simulink model "CartPendReal"  (R2015a)
settings: Solver=ode5  SolverMode=SingleTasking  StartTime=0.0  StopTime=inf  FixedStep=Ts  RelTol=1e-3  AbsTol=1e-6
values from neighbouring files (symbols this model uses):
  g = 9.81    [CartPendParams.mat]
  Jp = 0.00800173441225    [CartPendParams.mat]
  lpo = 0.20854    [CartPendParams.mat]
  lpwo = 0.455840449763    [CartPendParams.mat]
  mps = 0.0417185657763    [CartPendParams.mat]
  mpw = 0.0272036144897    [CartPendParams.mat]
  Ts = 0.01    [CartPendParams.mat]
  x0 = [0 3.14159265359 0 0]    [CartPendParams.mat]
undefined symbols (not defined in the file or in its folder): B1, B2, K, W1, W2
undefined symbols (not defined in the file): RTDAC4PCIBaseAddress
libraries: simulink x1
settings Model: SimulationMode=external  CovHtmlReporting=off  ExtModeTrigDuration=12000  ExtModeTrigLevel=0.400000  Creator=jims  LastModifiedBy=Student
settings DataIOCC: ExternalInput=[]  InitialState=[]  LimitDataPoints=off  MaxDataPoints=5000  SignalLoggingSaveFormat=ModelDataLogs  SaveOutput=off  SaveTime=off  SignalLoggingName=sigsOut
settings OptimizationCC: BooleanDataType=off  ExpressionDepthLimit=2147483647  InitFltsAndDblsToZero=on
settings DebuggingCC: SaveWithParameterizedLinksMsg=none  UnderspecifiedInitializationDetection=Classic  MergeDetectMultiDrivingBlocksExec=none  SignalResolutionControl=TryResolveAllWithWarning  MultiTaskDSMMsg=warning  MultiTaskCondExecSysMsg=none  IntegerOverflowMsg=none  FcnCallInpInsideContextMsg=EnableAllAsWarning  StateNameClashWarn=warning  IntegerSaturationMsg=none
settings HardwareCC: ProdBitPerLong=64  ProdBitPerPointer=64  ProdIntDivRoundTo=Zero  ProdEndianess=LittleEndian  ProdWordSize=64  ProdHWDeviceType=Intel->x86-64  TargetBitPerLong=64  TargetBitPerPointer=64  TargetIntDivRoundTo=Zero  TargetEndianess=LittleEndian  TargetWordSize=64  TargetHWDeviceType=Intel->x86-64
settings RTWCC: SystemTargetFile=rtwin.tlc  TemplateMakefile=RTDAC_win.tmf  Description=Real-Time Windows Target
settings RTWinTargetCC: TargetFcnLib=ansi_tfl_tmw.mat  TargetPreCompLibLocation=C:\Program Files\MATLAB\R2015aSP1\toolbox\sldrt\lib\win64  ModelReferenceCompliant=off  CompOptLevelCompliant=off

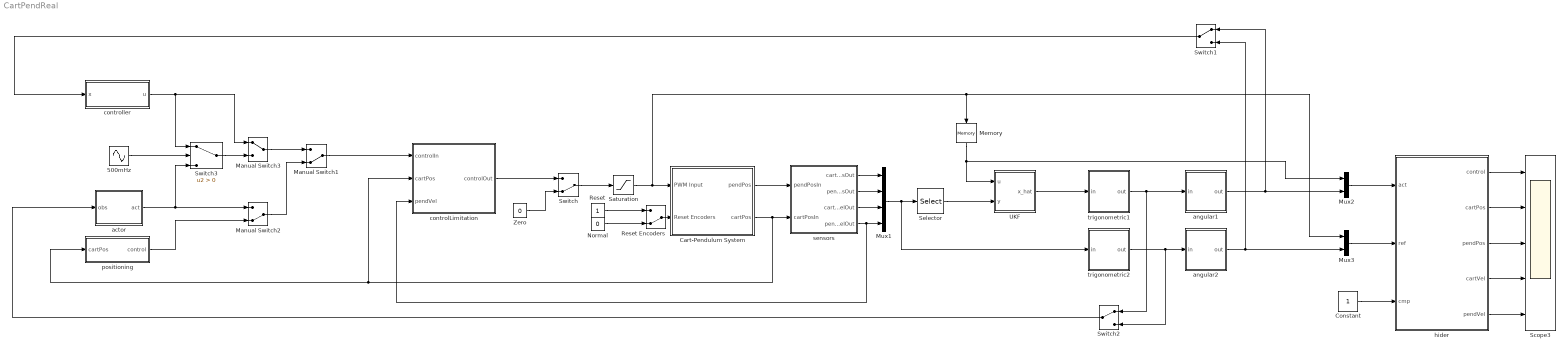
== system CartPendReal ==
  500mHz : Sin  Frequency=pi  SampleTime=Ts
  Cart-Pendulum System : Subsystem  mask{BaseAddress=RTDAC4PCIBaseAddress(-1,-1), T0=Ts}
      mask prompts: BaseAddress "Base Address:"; T0 "Sampling Period:"
      mask Display: plot( [0.725 0.725], [1.05 0.375], 0.725+0.05*sin([0:0.5:7]), 0.325+0.05*cos([0:0.5:7]), [-0.3 -0.3], [-0.3 -0.3], [1.8 1.8], [1.8 1.8], [0.1 1.4], [0.95 0.95], [0.1 1.4], [0.92 0.92], [0.65 0.8], [1 1], [0.65 0.8], [1.1 1.1], [0.65 0.65], [1.1 1], [0.8 0.8], [1 1.1] )
  Constant : Constant
  Manual Switch1 : ManualSwitch  CurrentSetting=0
  Manual Switch2 : ManualSwitch  CurrentSetting=0
  Manual Switch3 : ManualSwitch
  Memory : Memory
  Mux1 : Mux
  Mux2 : Mux  Inputs=2
  Mux3 : Mux  Inputs=2
  Normal : Constant  Value=0
  Reset : Constant
  Reset Encoders : ManualSwitch  CurrentSetting=0
  Saturation : Saturate
  Scope3 : Scope  NumInputPorts=5
      settings: TimeRange=15  YMin=-0.6~-1~-3.141592653589793~-5~-12  YMax=0.6~1~3.141592653589793~5~12  SampleInput=on  SampleTime=Ts  ScrollMode=on
  Selector : Selector  InputPortWidth=4  Indices=[1 2]
  Switch : ManualSwitch  CurrentSetting=0
  Switch1 : ManualSwitch
  Switch2 : ManualSwitch
  Switch3 : Switch  Criteria=u2 > Threshold
  UKF : Subsystem
  Zero : Constant  Value=0
  actor : MATLAB Function  TreatAsAtomicUnit=on  SystemSampleTime=Ts
  angular1 : Subsystem
  angular2 : Subsystem
  controlLimitation : Subsystem
  controller : Subsystem
  hider : Subsystem
  positioning : Subsystem
  sensors : Subsystem  mask(PENDULUM Output){T0=Ts}
      mask prompts: T0 "Sample Time"
      mask help: PCL-812 PG Device Driver
  trigonometric1 : Subsystem
  trigonometric2 : Subsystem
  wires:
  actor/1(act) -> Manual Switch2/1, Switch3/3
  Switch/1 -> Saturation/1
  Reset Encoders/1 -> Cart-Pendulum System/2(Reset Encoders)
  Reset/1 -> Reset Encoders/1
  Normal/1 -> Reset Encoders/2
  sensors/4(pendVelOut) -> Mux1/4, controlLimitation/3(pendVel)
  sensors/1(cartPosOut) -> Mux1/1
  sensors/2(pendPosOut) -> Mux1/2
  sensors/3(cartVelOut) -> Mux1/3
  Constant/1 -> hider/3(cmp)
  Zero/1 -> Switch/2
  Saturation/1 -> Memory/1, Mux3/1, Cart-Pendulum System/1(PWM Input)
  Mux1/1 -> Selector/1, trigonometric2/1(in)
  hider/5(pendVel) -> Scope3/5
  Selector/1 -> UKF/2(y)
  Mux3/1 -> hider/2(ref)
  Mux2/1 -> hider/1(act)
  UKF/1(x_hat) -> trigonometric1/1(in)
  Cart-Pendulum System/1(pendPos) -> sensors/1(pendPosIn)
  trigonometric1/1(out) -> angular1/1(in), Switch2/1
  trigonometric2/1(out) -> Switch2/2, angular2/1(in)
  positioning/1(control) -> Manual Switch2/2
  Manual Switch2/1 -> Manual Switch1/2
  controller/1(u) -> Manual Switch3/1, Switch3/1
  angular1/1(out) -> Mux2/2, Switch1/1
  angular2/1(out) -> Switch1/2, Mux3/2
  hider/1(control) -> Scope3/1
  hider/2(cartPos) -> Scope3/2
  hider/3(pendPos) -> Scope3/3
  hider/4(cartVel) -> Scope3/4
  500mHz/1 -> Switch3/2
  Switch3/1 -> Manual Switch3/2
  Switch2/1 -> actor/1(obs)
  Manual Switch3/1 -> Manual Switch1/1
  Memory/1 -> UKF/1(u), Mux2/1
  controlLimitation/1(controlOut) -> Switch/1
  Cart-Pendulum System/2(cartPos) -> controlLimitation/2(cartPos), positioning/1(cartPos), sensors/2(cartPosIn)
  Switch1/1 -> controller/1(x)
  Manual Switch1/1 -> controlLimitation/1(controlIn)

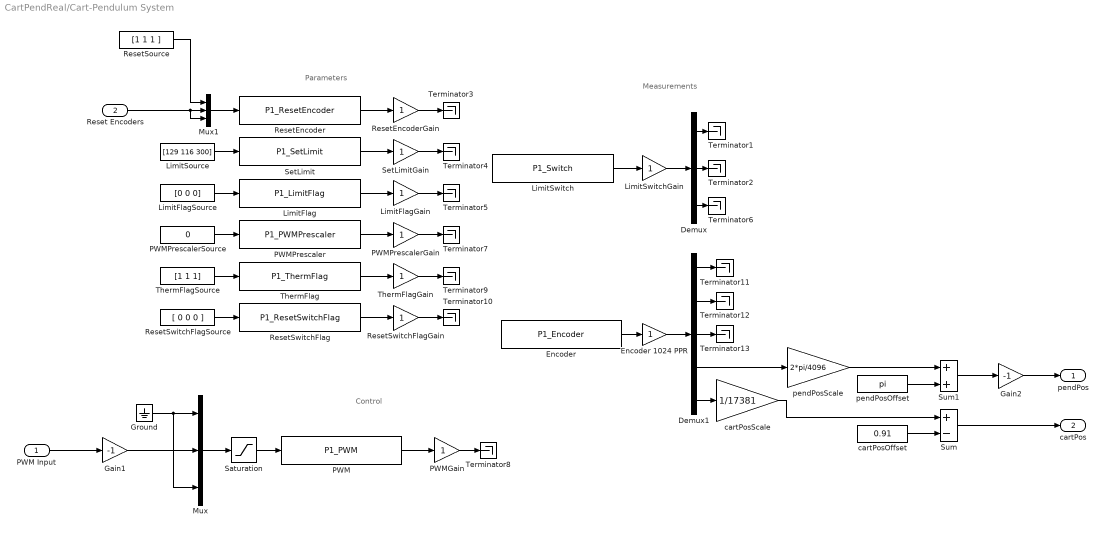
== system CartPendReal/Cart-Pendulum System ==
  note: Measurements
  note: Control
  note: Parameters
  PWM Input : Inport
  Reset Encoders : Inport  Port=2
  Demux : Demux  Outputs=3
  Demux1 : Demux  Outputs=5
  Encoder : S-Function  FunctionName=P1_Encoder  Parameters=BaseAddress, T0
  Encoder 1024 PPR : Gain  SaturateOnIntegerOverflow=on  OutDataTypeStr=Inherit: Same as input  ParamDataTypeStr=Inherit: Same as input
  Gain1 : Gain  Gain=-1
  Gain2 : Gain  Gain=-1
  Ground : Ground
  LimitFlag : S-Function  FunctionName=P1_LimitFlag  Parameters=BaseAddress, T0
  LimitFlagGain : Gain  SaturateOnIntegerOverflow=on  OutDataTypeStr=Inherit: Same as input  ParamDataTypeStr=Inherit: Same as input
  LimitFlagSource : Constant  Value=[0 0 0]
  LimitSource : Constant  Value=[129 116 300]
  LimitSwitch : S-Function  FunctionName=P1_Switch  Parameters=BaseAddress, T0
  LimitSwitchGain : Gain  SaturateOnIntegerOverflow=on  OutDataTypeStr=Inherit: Same as input  ParamDataTypeStr=Inherit: Same as input
  Mux : Mux  Inputs=3
  Mux1 : Mux  Inputs=[3 1 1]
  PWM : S-Function  FunctionName=P1_PWM  Parameters=BaseAddress, T0
  PWMGain : Gain  SaturateOnIntegerOverflow=on  OutDataTypeStr=Inherit: Same as input  ParamDataTypeStr=Inherit: Same as input
  PWMPrescaler : S-Function  FunctionName=P1_PWMPrescaler  Parameters=BaseAddress, T0
  PWMPrescalerGain : Gain  SaturateOnIntegerOverflow=on  OutDataTypeStr=Inherit: Same as input  ParamDataTypeStr=Inherit: Same as input
  PWMPrescalerSource : Constant  Value=0
  ResetEncoder : S-Function  FunctionName=P1_ResetEncoder  Parameters=BaseAddress, T0
  ResetEncoderGain : Gain  SaturateOnIntegerOverflow=on  OutDataTypeStr=Inherit: Same as input  ParamDataTypeStr=Inherit: Same as input
  ResetSource : Constant  Value=[1 1 1 ]
  "ResetSwitchFlag " : S-Function  FunctionName=P1_ResetSwitchFlag  Parameters=BaseAddress, T0
  ResetSwitchFlagGain : Gain  SaturateOnIntegerOverflow=on  OutDataTypeStr=Inherit: Same as input  ParamDataTypeStr=Inherit: Same as input
  ResetSwitchFlagSource : Constant  Value=[ 0 0 0 ]
  Saturation : Saturate
  SetLimit : S-Function  FunctionName=P1_SetLimit  Parameters=BaseAddress, T0
  SetLimitGain : Gain  SaturateOnIntegerOverflow=on  OutDataTypeStr=Inherit: Same as input  ParamDataTypeStr=Inherit: Same as input
  Sum : Sum  Inputs=+-  SaturateOnIntegerOverflow=on  InputSameDT=on  OutDataTypeStr=Inherit: Same as first input
  Sum1 : Sum  SaturateOnIntegerOverflow=on  InputSameDT=on  OutDataTypeStr=Inherit: Same as first input
  Terminator{1..13} (13 alike) : Terminator
  "ThermFlag " : S-Function  FunctionName=P1_ThermFlag  Parameters=BaseAddress, T0
  ThermFlagGain : Gain  SaturateOnIntegerOverflow=on  OutDataTypeStr=Inherit: Same as input  ParamDataTypeStr=Inherit: Same as input
  ThermFlagSource : Constant  Value=[1 1 1]
  cartPosOffset : Constant  Value=0.91
  cartPosScale : Gain  Gain=1/17381  OutDataTypeStr=Inherit: Same as input  ParamDataTypeStr=Inherit: Same as input
  pendPosOffset : Constant  Value=pi
  pendPosScale : Gain  Gain=2*pi/4096  OutDataTypeStr=Inherit: Same as input  ParamDataTypeStr=Inherit: Same as input
  pendPos : Outport
  cartPos : Outport  Port=2
  wires:
  Demux1/1 -> Terminator11/1
  Demux1/2 -> Terminator12/1
  Demux1/3 -> Terminator13/1
  Demux/3 -> Terminator6/1
  Demux/2 -> Terminator2/1
  Demux/1 -> Terminator1/1
  LimitSwitchGain/1 -> Demux/1
  LimitSwitch/1 -> LimitSwitchGain/1
  Ground/1 -> Mux/1, Mux/3
  PWM Input/1 -> Gain1/1
  ResetSwitchFlagGain/1 -> Terminator10/1
  ThermFlagGain/1 -> Terminator9/1
  PWMPrescalerGain/1 -> Terminator7/1
  LimitFlagGain/1 -> Terminator5/1
  SetLimitGain/1 -> Terminator4/1
  ResetEncoderGain/1 -> Terminator3/1
  ResetSwitchFlagSource/1 -> "ResetSwitchFlag "/1
  ThermFlagSource/1 -> "ThermFlag "/1
  PWMPrescalerSource/1 -> PWMPrescaler/1
  LimitFlagSource/1 -> LimitFlag/1
  LimitSource/1 -> SetLimit/1
  "ResetSwitchFlag "/1 -> ResetSwitchFlagGain/1
  "ThermFlag "/1 -> ThermFlagGain/1
  PWMPrescaler/1 -> PWMPrescalerGain/1
  LimitFlag/1 -> LimitFlagGain/1
  SetLimit/1 -> SetLimitGain/1
  ResetEncoder/1 -> ResetEncoderGain/1
  PWMGain/1 -> Terminator8/1
  PWM/1 -> PWMGain/1
  Mux/1 -> Saturation/1
  Saturation/1 -> PWM/1
  Encoder/1 -> Encoder 1024 PPR/1
  Encoder 1024 PPR/1 -> Demux1/1
  Mux1/1 -> ResetEncoder/1
  ResetSource/1 -> Mux1/1
  Reset Encoders/1 -> Mux1/2, Mux1/3
  pendPosScale/1 -> Sum1/1
  pendPosOffset/1 -> Sum1/2
  Gain1/1 -> Mux/2
  Sum1/1 -> Gain2/1
  Sum/1 -> cartPos/1
  Demux1/4 -> pendPosScale/1
  Gain2/1 -> pendPos/1
  Demux1/5 -> cartPosScale/1
  cartPosOffset/1 -> Sum/2
  cartPosScale/1 -> Sum/1

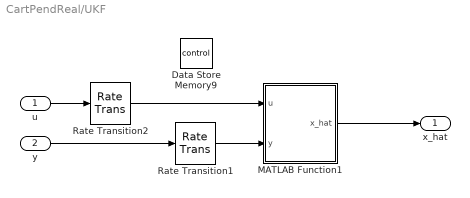
== system CartPendReal/UKF ==
  u : Inport
  y : Inport  Port=2
  Data Store Memory9 : DataStoreMemory  DataStoreName=control  ReadBeforeWriteMsg=warning  WriteAfterWriteMsg=warning  WriteAfterReadMsg=warning  OutDataTypeStr=double
  MATLAB Function1 : MATLAB Function  TreatAsAtomicUnit=on
  Rate Transition1 : RateTransition  X0=x0(1:2)  OutPortSampleTime=Ts
  Rate Transition2 : RateTransition  OutPortSampleTime=Ts
  x_hat : Outport
  wires:
  Rate Transition2/1 -> MATLAB Function1/1(u)
  Rate Transition1/1 -> MATLAB Function1/2(y)
  y/1 -> Rate Transition1/1
  MATLAB Function1/1(x_hat) -> x_hat/1
  u/1 -> Rate Transition2/1

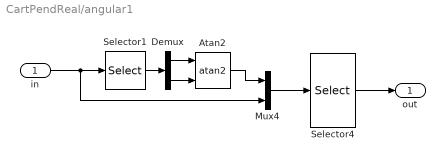
== system CartPendReal/angular1 ==
  in : Inport
  Atan2 : Trigonometry  Operator=atan2
  Demux : Demux  Outputs=2
  Mux4 : Mux  Inputs=2
  Selector1 : Selector  InputPortWidth=5  Indices=[2 3]
  Selector4 : Selector  InputPortWidth=6  Indices=[2 1 5 6]
  out : Outport
  wires:
  Demux/2 -> Atan2/2
  in/1 -> Mux4/2, Selector1/1
  Atan2/1 -> Mux4/1
  Demux/1 -> Atan2/1
  Mux4/1 -> Selector4/1
  Selector4/1 -> out/1
  Selector1/1 -> Demux/1

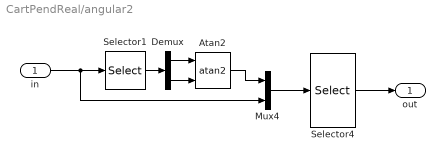
== system CartPendReal/angular2 ==
  in : Inport
  Atan2 : Trigonometry  Operator=atan2
  Demux : Demux  Outputs=2
  Mux4 : Mux  Inputs=2
  Selector1 : Selector  InputPortWidth=5  Indices=[2 3]
  Selector4 : Selector  InputPortWidth=6  Indices=[2 1 5 6]
  out : Outport
  wires:
  Demux/2 -> Atan2/2
  in/1 -> Mux4/2, Selector1/1
  Atan2/1 -> Mux4/1
  Demux/1 -> Atan2/1
  Mux4/1 -> Selector4/1
  Selector4/1 -> out/1
  Selector1/1 -> Demux/1

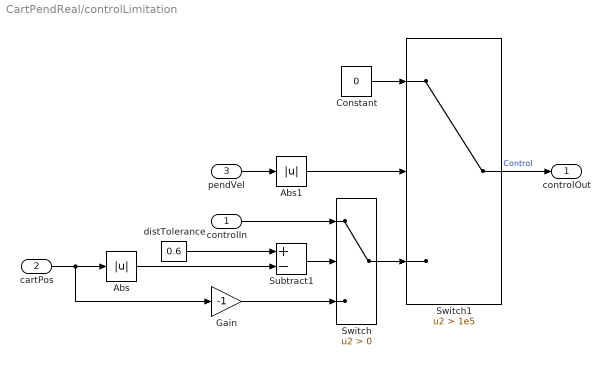
== system CartPendReal/controlLimitation ==
  controlIn : Inport
  cartPos : Inport  Port=2
  pendVel : Inport  Port=3
  Abs : Abs
  Abs1 : Abs
  Constant : Constant  Value=0
  Gain : Gain  Gain=-1
  Subtract1 : Sum  Inputs=+-
  Switch : Switch  Criteria=u2 > Threshold
  Switch1 : Switch  Criteria=u2 > Threshold  Threshold=1e5
  distTolerance : Constant  Value=0.6
  controlOut : Outport
  wires:
  controlIn/1 -> Switch/1
  distTolerance/1 -> Subtract1/1
  Switch1/1 -> controlOut/1  "Control"
  Subtract1/1 -> Switch/2
  Abs/1 -> Subtract1/2
  cartPos/1 -> Abs/1, Gain/1
  Gain/1 -> Switch/3
  pendVel/1 -> Abs1/1
  Abs1/1 -> Switch1/2
  Constant/1 -> Switch1/1
  Switch/1 -> Switch1/3

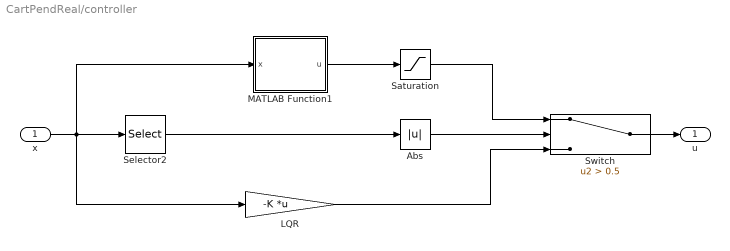
== system CartPendReal/controller ==
  x : Inport
  Abs : Abs
  LQR : Gain  Gain=-K  Multiplication=Matrix(K*u) (u vector)
  MATLAB Function1 : MATLAB Function  TreatAsAtomicUnit=on  SystemSampleTime=Ts
  Saturation : Saturate  UpperLimit=0.4  LowerLimit=-0.4
  Selector2 : Selector  InputPortWidth=4  Indices=[2]
  Switch : Switch  Criteria=u2 > Threshold  Threshold=0.5
  u : Outport
  wires:
  MATLAB Function1/1(u) -> Saturation/1
  Selector2/1 -> Abs/1
  Abs/1 -> Switch/2
  Switch/1 -> u/1
  x/1 -> LQR/1, Selector2/1, MATLAB Function1/1(x)
  LQR/1 -> Switch/3
  Saturation/1 -> Switch/1

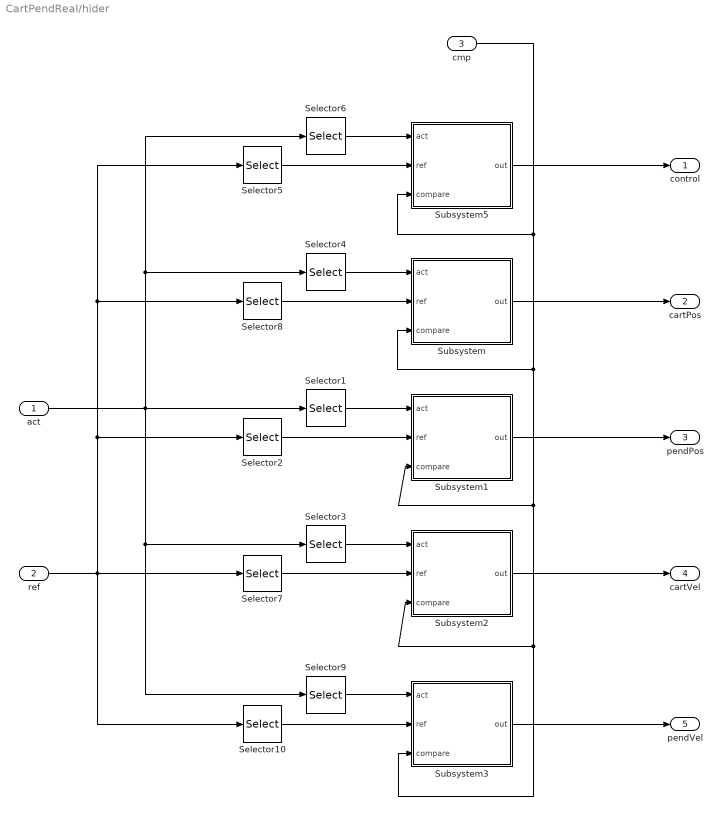
== system CartPendReal/hider ==
  act : Inport
  ref : Inport  Port=2
  cmp : Inport  Port=3
  Selector1 : Selector  InputPortWidth=5  Indices=[3]
  Selector10 : Selector  InputPortWidth=5  Indices=[5]
  Selector2 : Selector  InputPortWidth=5  Indices=[3]
  Selector3 : Selector  InputPortWidth=5  Indices=[4]
  Selector4 : Selector  InputPortWidth=5  Indices=[2]
  Selector5 : Selector  InputPortWidth=5  Indices=[1]
  Selector6 : Selector  InputPortWidth=5  Indices=[1]
  Selector7 : Selector  InputPortWidth=5  Indices=[4]
  Selector8 : Selector  InputPortWidth=5  Indices=[2]
  Selector9 : Selector  InputPortWidth=5  Indices=[5]
  Subsystem : Subsystem
  Subsystem1 : Subsystem
  Subsystem2 : Subsystem
  Subsystem3 : Subsystem
  Subsystem5 : Subsystem
  control : Outport
  cartPos : Outport  Port=2
  pendPos : Outport  Port=3
  cartVel : Outport  Port=4
  pendVel : Outport  Port=5
  wires:
  Selector8/1 -> Subsystem/2(ref)
  Selector4/1 -> Subsystem/1(act)
  Subsystem/1(out) -> cartPos/1
  Selector2/1 -> Subsystem1/2(ref)
  Selector1/1 -> Subsystem1/1(act)
  Subsystem1/1(out) -> pendPos/1
  Selector7/1 -> Subsystem2/2(ref)
  Selector3/1 -> Subsystem2/1(act)
  Subsystem2/1(out) -> cartVel/1
  Selector10/1 -> Subsystem3/2(ref)
  Selector9/1 -> Subsystem3/1(act)
  Subsystem3/1(out) -> pendVel/1
  Selector5/1 -> Subsystem5/2(ref)
  Subsystem5/1(out) -> control/1
  act/1 -> Selector9/1, Selector3/1, Selector1/1, Selector6/1, Selector4/1
  Selector6/1 -> Subsystem5/1(act)
  cmp/1 -> Subsystem2/3(compare), Subsystem3/3(compare), Subsystem1/3(compare), Subsystem/3(compare), Subsystem5/3(compare)
  ref/1 -> Selector10/1, Selector7/1, Selector2/1, Selector5/1, Selector8/1

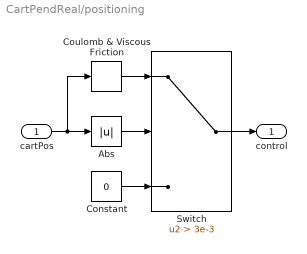
== system CartPendReal/positioning ==
  cartPos : Inport
  Abs : Abs
  Constant : Constant  Value=0
  Coulomb & Viscous Friction : simulink/Discontinuities/Coulomb & Viscous Friction  offset=-0.1  gain=-1
  Switch : Switch  Criteria=u2 > Threshold  Threshold=3e-3
  control : Outport
  wires:
  cartPos/1 -> Coulomb & Viscous Friction/1, Abs/1
  Switch/1 -> control/1
  Abs/1 -> Switch/2
  Coulomb & Viscous Friction/1 -> Switch/1
  Constant/1 -> Switch/3

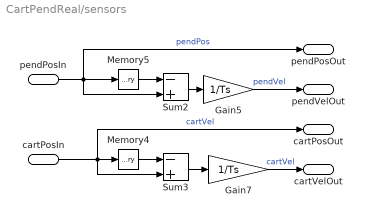
== system CartPendReal/sensors ==
  pendPosIn : Inport
  cartPosIn : Inport  Port=2
  Gain5 : Gain  Gain=1/Ts  SaturateOnIntegerOverflow=on  OutDataTypeStr=Inherit: Same as input  ParamDataTypeStr=Inherit: Same as input
  Gain7 : Gain  Gain=1/Ts  SaturateOnIntegerOverflow=on  OutDataTypeStr=Inherit: Same as input  ParamDataTypeStr=Inherit: Same as input
  Memory4 : Memory  X0=x0(1)
  Memory5 : Memory  X0=x0(2)
  Sum2 : Sum  Inputs=-+  SaturateOnIntegerOverflow=on  InputSameDT=on  OutDataTypeStr=Inherit: Same as first input
  Sum3 : Sum  Inputs=-+  SaturateOnIntegerOverflow=on  InputSameDT=on  OutDataTypeStr=Inherit: Same as first input
  cartPosOut : Outport  InitialOutput=0
  pendPosOut : Outport  Port=2  InitialOutput=0
  cartVelOut : Outport  Port=3  InitialOutput=0
  pendVelOut : Outport  Port=4  InitialOutput=0
  wires:
  cartPosIn/1 -> Sum3/2, cartPosOut/1, Memory4/1  "cartVel"
  Gain5/1 -> pendVelOut/1  "pendVel"
  pendPosIn/1 -> pendPosOut/1, Sum2/2, Memory5/1  "pendPos"
  Gain7/1 -> cartVelOut/1  "cartVel"
  Sum3/1 -> Gain7/1
  Memory5/1 -> Sum2/1
  Memory4/1 -> Sum3/1
  Sum2/1 -> Gain5/1

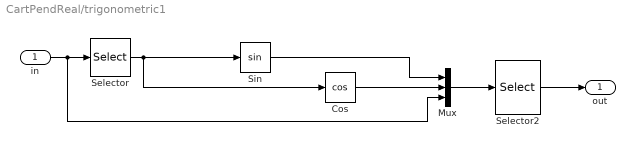
== system CartPendReal/trigonometric1 ==
  in : Inport
  Cos : Trigonometry  Operator=cos
  Mux : Mux  Inputs=3
  Selector : Selector  InputPortWidth=4  Indices=2
  Selector2 : Selector  InputPortWidth=6  Indices=[3 1 2 5 6]
  Sin : Trigonometry
  out : Outport
  wires:
  Sin/1 -> Mux/1
  Cos/1 -> Mux/2
  Selector/1 -> Sin/1, Cos/1
  in/1 -> Mux/3, Selector/1
  Mux/1 -> Selector2/1
  Selector2/1 -> out/1

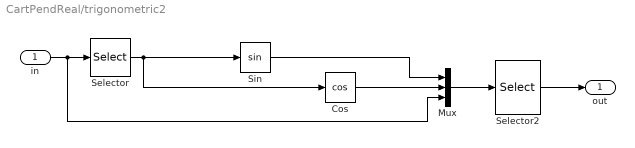
== system CartPendReal/trigonometric2 ==
  in : Inport
  Cos : Trigonometry  Operator=cos
  Mux : Mux  Inputs=3
  Selector : Selector  InputPortWidth=4  Indices=2
  Selector2 : Selector  InputPortWidth=6  Indices=[3 1 2 5 6]
  Sin : Trigonometry
  out : Outport
  wires:
  Sin/1 -> Mux/1
  Cos/1 -> Mux/2
  Selector/1 -> Sin/1, Cos/1
  in/1 -> Mux/3, Selector/1
  Mux/1 -> Selector2/1
  Selector2/1 -> out/1

== system CartPendReal/hider/Subsystem ==
  act : Inport
  ref : Inport  Port=2
  compare : Inport  Port=3
  Mux1 : Mux  Inputs=2
  Switch : Switch  Criteria=u2 > Threshold
  out : Outport
  wires:
  compare/1 -> Switch/2
  Switch/1 -> out/1
  Mux1/1 -> Switch/1
  ref/1 -> Mux1/1
  act/1 -> Mux1/2, Switch/3

== system CartPendReal/hider/Subsystem1 ==
  act : Inport
  ref : Inport  Port=2
  compare : Inport  Port=3
  Mux1 : Mux  Inputs=2
  Switch : Switch  Criteria=u2 > Threshold
  out : Outport
  wires:
  compare/1 -> Switch/2
  Switch/1 -> out/1
  Mux1/1 -> Switch/1
  ref/1 -> Mux1/1
  act/1 -> Mux1/2, Switch/3

== system CartPendReal/hider/Subsystem2 ==
  act : Inport
  ref : Inport  Port=2
  compare : Inport  Port=3
  Mux1 : Mux  Inputs=2
  Switch : Switch  Criteria=u2 > Threshold
  out : Outport
  wires:
  compare/1 -> Switch/2
  Switch/1 -> out/1
  Mux1/1 -> Switch/1
  ref/1 -> Mux1/1
  act/1 -> Mux1/2, Switch/3

== system CartPendReal/hider/Subsystem3 ==
  act : Inport
  ref : Inport  Port=2
  compare : Inport  Port=3
  Mux1 : Mux  Inputs=2
  Switch : Switch  Criteria=u2 > Threshold
  out : Outport
  wires:
  compare/1 -> Switch/2
  Switch/1 -> out/1
  Mux1/1 -> Switch/1
  ref/1 -> Mux1/1
  act/1 -> Mux1/2, Switch/3

== system CartPendReal/hider/Subsystem5 ==
  act : Inport
  ref : Inport  Port=2
  compare : Inport  Port=3
  Mux1 : Mux  Inputs=2
  Switch : Switch  Criteria=u2 > Threshold
  out : Outport
  wires:
  compare/1 -> Switch/2
  Switch/1 -> out/1
  Mux1/1 -> Switch/1
  ref/1 -> Mux1/1
  act/1 -> Mux1/2, Switch/3

== matlab function CartPendReal/controller/MATLAB Function1 ==
  data: x input size=4; u output; mpw parameter; mps parameter; lpwo parameter; lpo parameter; g parameter; Jp parameter
function u = swingUp(x, mpw, mps, lpwo, lpo, g, Jp)
cartPos = x(1);
pendPos = x(2);
pendVel = x(4);
Ep = (mpw*lpwo + mps*lpo)*g*(cos(pendPos) + 1);
Ek = (Jp*pendVel^2)/2;
Em = Ep + Ek;
Emtop = 2*g*(mpw*lpwo + mps*lpo);
if (Em < Emtop)
    u = sign(pendVel*cos(pendPos))/2 - cartPos;
else
    u = 0;
end

== matlab function CartPendReal/actor ==
  data: obs input size=5; act output size=1; W1 parameter; B1 parameter; W2 parameter; B2 parameter
function act = policy(obs, W1, B1, W2, B2)
    u = max(0, W1*obs + B1);
    u = tanh(W2*u + B2);
    u = max(-0.5, 0.5*u);
    u = min(u, 0.5);
    act = double(u);
end

== matlab function CartPendReal/UKF/MATLAB Function1 ==
  data: u input size=1; x_hat output size=4; y input size=2; control data_store_memory
function x_hat = UKF(u, y)
  global control
  control = u;
  persistent P x
  if isempty(P)
    P = eye(4);
  end
  if isempty(x)
    x = [0 pi 0 0]';
  end
  Ts = 0.01;
  f = @CartPendStep;
  h = @CartPendOut;
  z = y;
  Q = diag([1/17381 2*pi/4096 1/17381/Ts 2*pi/4096/Ts])^2;
  R = diag([0 20*pi/4096])^2;
  [x, P] = ukf(f, x, P, h, z, Q, R);
  x_hat = x;
end

function x_out = CartPendOut(x)
  x_out = x(1:2);
end

function y_out = CartPendStep(x)
  Ts = 0.01;
  [~, y] = ode45(@CartPendDeriv, [0 Ts 2*Ts], x);
  y_out = y(2, :)';
end

function xdot = CartPendDeriv(~, x)
  global control

  fs = 0.324838868217633;
  fc = 2.099102042804786;
  fp = 8.000000082571058e-04;
  p1 = 19.442829589021017;
  p2 = -1.263717424289592;
  m = 0.999999999999989;
  l = 0.019100377624366;
  g = 9.81;
  Jp = 0.008001734412250;

  u = max(-0.5, min(control, 0.5));
  u = abs(abs(fs/p1) - abs(u));
  u = (u > abs(fs/p1))*sign(control)*u;

  x1dot = x(3);
  x2dot = x(4);

  horz = l*sin(x(2));
  vert = l*cos(x(2));
  torq = m*g*horz - fp*x2dot;
  force = x1dot*(fc - p2) + m*horz*x2dot^2 - p1*u;
  div = Jp - m*vert^2;

  x1ddot = (torq*vert - force*Jp/m)/div; % cart acc
  x2ddot = (torq - force*vert)/div; % pend acc

  x3dot = x1ddot;
  x4dot = x2ddot;

  xdot = [x1dot x2dot x3dot x4dot]'; % d/dt[x, 0, v, w]
end
